simulink model "simulink_13"  (R2023b)
settings: Solver=FixedStepAuto  StartTime=0.0  StopTime=10.0  FixedStep=0.001  RelTol=1e-3
libraries: simulink x1
(part 1 of 3)
settings Model: Creator=Carlo  LastModifiedBy=Carlo

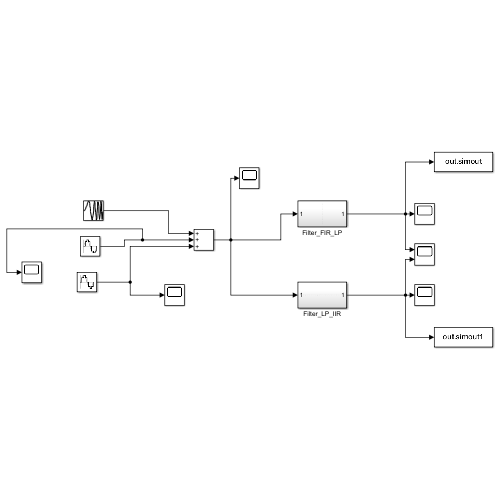
[thumbnail: Simulink's stored preview of the top-level diagram]
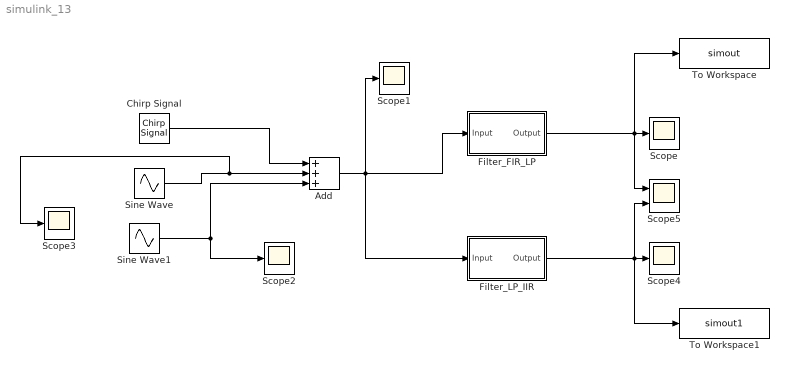
== system simulink_13 ==
  Add : Sum  Inputs=+++
  Chirp Signal : simulink/Sources/Chirp Signal  f1=10  T=10  f2=100
  Filter_FIR_LP : Subsystem  Tag=FilterWizardSubSystem
      settings: ErrorFcn=dspFilterRealizedInBasicElemsAlgLoopErrFcnCallback
  Filter_LP_IIR : Subsystem  Tag=FilterWizardSubSystem
      settings: ErrorFcn=dspFilterRealizedInBasicElemsAlgLoopErrFcnCallback
  Scope{,1..4} (5 alike) : Scope
  Scope5 : Scope  NumInputPorts=2
  Sine Wave : Sin  Amplitude=2  Frequency=30*(2*3.14)  SampleTime=0.001
  Sine Wave1 : Sin  Frequency=75*3.14  SampleTime=0.001
  To Workspace : ToWorkspace  VariableName=simout  SaveFormat=Timeseries  SampleTime=-1
  To Workspace1 : ToWorkspace  VariableName=simout1  SaveFormat=Timeseries  SampleTime=-1
  wires:
  Sine Wave1/1 -> Add/3, Scope2/1
  Sine Wave/1 -> Scope3/1, Add/2
  Filter_FIR_LP/1(Output) -> To Workspace/1, Scope5/1, Scope/1
  Add/1 -> Filter_LP_IIR/1(Input), Filter_FIR_LP/1(Input), Scope1/1
  Chirp Signal/1 -> Add/1
  Filter_LP_IIR/1(Output) -> Scope5/2, Scope4/1, To Workspace1/1
